simulink model "ProdSys_MakeToStockPULL_CONWIP"  (R2015a)
settings: Solver=ode45  SolverMode=SingleTasking  StartTime=0.0  StopTime=10.0  RelTol=1e-3
undefined symbols (not defined in the file or in its folder): se_randomizeseeds
libraries: simeventslib x10, simulink x1
(part 1 of 2)
settings Model: CovSFcnEnable=off  Creator=AnotherUser  LastModifiedBy=gthiers3
settings OptimizationCC: BlockReduction=off  BooleanDataType=off
settings DebuggingCC: SaveWithParameterizedLinksMsg=none  UnderspecifiedInitializationDetection=Classic  MergeDetectMultiDrivingBlocksExec=none  SignalResolutionControl=TryResolveAllWithWarning  StrictBusMsg=Warning
settings HardwareCC: TargetUnknown=on

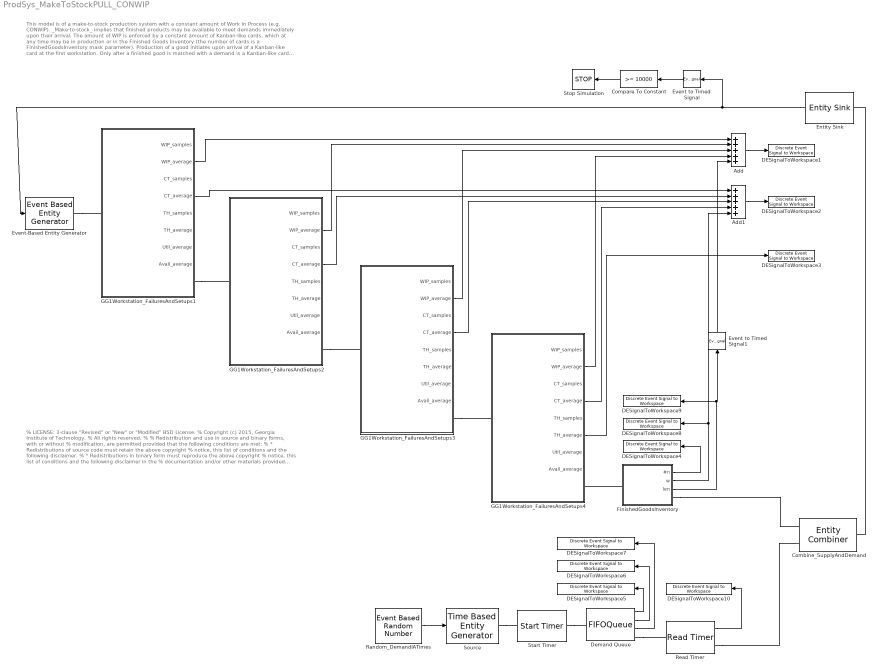
== system ProdSys_MakeToStockPULL_CONWIP ==
  note: This model is of a make-to-stock production system with a constant amount of Work In Process (e.g. CONWIP).
      | _Make-to-stock_ implies that finished products may be available to meet demands immediately upon their arrival.
      | The amount of WIP is enforced by a constant amount of Kanban-like cards, which at any time may be in production
      | or in the Finished Goods Inventory (the number of cards is a FinishedGoodsInventory mask parameter). Production
      | of a good initiates upon arrival of a Kanban-like card at the first workstation.  Only after a finished good is matched
      | with a demand is a Kanban-like card freed and recycled through a feedback loop.
      |
      | NOTE that each GG1Workstation_FailuresAndSetups# is a usage of a block in the SingleWorkstationModelLibrary,
      | and that library may need to be accessible on MATLAB's path.
  note: % LICENSE: 3-clause "Revised" or "New" or "Modified" BSD License.
      | % Copyright (c) 2015, Georgia Institute of Technology.
      | % All rights reserved.
      | %
      | % Redistribution and use in source and binary forms, with or without
      | % modification, are permitted provided that the following conditions are met:
      | % * Redistributions of source code must retain the above copyright
      | % notice, this list of conditions and the following disclaimer.
      | % * Redistributions in binary form must reproduce the above copyright
      | % notice, this list of conditions and the following disclaimer in the
      | % documentation and/or other materials provided with the distribution.
      | % * Neither the name of the Georgia Institute of Technology nor the
      | % names of its contributors may be used to endorse or promote products
      | % derived from this software without specific prior written permission.
      | %
      | % THIS SOFTWARE IS PROVIDED BY THE COPYRIGHT HOLDERS AND CONTRIBUTORS "AS IS" AND
      | % ANY EXPRESS OR IMPLIED WARRANTIES, INCLUDING, BUT NOT LIMITED TO, THE IMPLIED
      | % WARRANTIES OF MERCHANTABILITY AND FITNESS FOR A PARTICULAR PURPOSE ARE
      | % DISCLAIMED. IN NO EVENT SHALL THE GEORGIA INSTITUTE OF TECHNOLOGY BE LIABLE FOR
      | % ANY DIRECT, INDIRECT, INCIDENTAL, SPECIAL, EXEMPLARY, OR CONSEQUENTIAL DAMAGES
      | % (INCLUDING, BUT NOT LIMITED TO, PROCUREMENT OF SUBSTITUTE GOODS OR SERVICES;
      | % LOSS OF USE, DATA, OR PROFITS; OR BUSINESS INTERRUPTION) HOWEVER CAUSED AND
      | % ON ANY THEORY OF LIABILITY, WHETHER IN CONTRACT, STRICT LIABILITY, OR TORT
      | % (INCLUDING NEGLIGENCE OR OTHERWISE) ARISING IN ANY WAY OUT OF THE USE OF THIS
      | % SOFTWARE, EVEN IF ADVISED OF THE POSSIBILITY OF SUCH DAMAGE.
  Add : Sum  Inputs=+++++
  Add1 : Sum  Inputs=+++++
  Combine_SupplyAndDemand : EntityCombiner  NumberInputPorts=2  RetainComponentEntities=off
  Compare To Constant : simulink/Logic and Bit Operations/Compare To Constant  relop=>=  const=10000  OutDataTypeStr=boolean
  DESignalToWorkspace1 : simeventslib/SimEvents Sinks/Discrete Event Signal to Workspace  VariableName=WIP_average  SaveFormat=Structure With Time  isMonitorOnly=off  isRecordIC=off
  DESignalToWorkspace10 : simeventslib/SimEvents Sinks/Discrete Event Signal to Workspace  VariableName=DemandWaitTimes  SaveFormat=Structure With Time  isMonitorOnly=off  isRecordIC=off
  DESignalToWorkspace2 : simeventslib/SimEvents Sinks/Discrete Event Signal to Workspace  VariableName=CT_average  SaveFormat=Structure With Time  isMonitorOnly=off  isRecordIC=off
  DESignalToWorkspace3 : simeventslib/SimEvents Sinks/Discrete Event Signal to Workspace  VariableName=TH_average  SaveFormat=Structure With Time  isMonitorOnly=off  isRecordIC=off
  DESignalToWorkspace4 : simeventslib/SimEvents Sinks/Discrete Event Signal to Workspace  VariableName=FGI_samples  SaveFormat=Structure With Time  isMonitorOnly=off  isRecordIC=off
  DESignalToWorkspace5 : simeventslib/SimEvents Sinks/Discrete Event Signal to Workspace  VariableName=Backorders_samples  SaveFormat=Structure With Time  isMonitorOnly=off  isRecordIC=off
  DESignalToWorkspace6 : simeventslib/SimEvents Sinks/Discrete Event Signal to Workspace  VariableName=Backorders_avgWait  SaveFormat=Structure With Time  isMonitorOnly=off  isRecordIC=off
  DESignalToWorkspace7 : simeventslib/SimEvents Sinks/Discrete Event Signal to Workspace  VariableName=Backorders_avgLen  SaveFormat=Structure With Time  isMonitorOnly=off  isRecordIC=off
  DESignalToWorkspace8 : simeventslib/SimEvents Sinks/Discrete Event Signal to Workspace  VariableName=FGI_avgWait  SaveFormat=Structure With Time  isMonitorOnly=off  isRecordIC=off
  DESignalToWorkspace9 : simeventslib/SimEvents Sinks/Discrete Event Signal to Workspace  VariableName=FGI_avgLen  SaveFormat=Structure With Time  isMonitorOnly=off  isRecordIC=off
  Demand Queue : FIFOQueue  Capacity=inf  StatNumberInBlock=on  StatAverageWait=on  StatAverageQueueLength=on
      settings: OutputPortMap=o1,o2,o3
  Entity Sink : EntitySink  StatNumberArrived=on
  Event to Timed Signal : EventToTimedSignal
  Event to Timed Signal1 : EventToTimedSignal
  Event-Based Entity Generator : EventBasedEntityGenerator  ResponseDuringBlockage=Delay first pending entity
  FinishedGoodsInventory : Subsystem  mask{NumberOfEventsPerPeriod=10}
      mask prompts: NumberOfEventsPerPeriod "Number of Kanban-like cards in the system:"
      mask TypeOptions NumberOfEventsPerPeriod: T0_FcnCallGen/NumberOfEventsPerPeriod
      mask DialogControl DescTextVar Prompt: Finished Goods Inventory:  Make-to-stock implies that finished goods may be produced in advance of demand arrivals.  This subsystem is effectively a queue, storing finished goods which have not yet been matched with demand.
  GG1Workstation_FailuresAndSetups1 : Subsystem  InitFcn=se_randomizeseeds(gcs, 'Mode', 'All')
      settings: CopyFcn=set_param(gcb, 'LinkStatus', 'none');
  GG1Workstation_FailuresAndSetups2 : Subsystem  InitFcn=se_randomizeseeds(gcs, 'Mode', 'All')
      settings: CopyFcn=set_param(gcb, 'LinkStatus', 'none');
  GG1Workstation_FailuresAndSetups3 : Subsystem  InitFcn=se_randomizeseeds(gcs, 'Mode', 'All')
      settings: CopyFcn=set_param(gcb, 'LinkStatus', 'none');
  GG1Workstation_FailuresAndSetups4 : Subsystem  InitFcn=se_randomizeseeds(gcs, 'Mode', 'All')
      settings: CopyFcn=set_param(gcb, 'LinkStatus', 'none');
  Random_DemandIATimes : EventBasedRandomNumber  Distribution=Gamma  scaleGam=2  shapeGam=10  meanNorm=100  stdNorm=eps  Seed=10339
  Read Timer : ReadTimer  StatTimeElapsed=on
      settings: OutputPortMap=o2
  Source : TimeBasedEntityGenerator  GenerateEntitiesUpon=Intergeneration time from port t
  Start Timer : StartTimer
  Stop Simulation : Stop
  wires:
  Random_DemandIATimes/1 -> Source/1
  Entity Sink/1 -> Event to Timed Signal/1, Event-Based Entity Generator/1
  Compare To Constant/1 -> Stop Simulation/1
  Event to Timed Signal/1 -> Compare To Constant/1
  GG1Workstation_FailuresAndSetups1/2(WIP_average) -> Add/1
  GG1Workstation_FailuresAndSetups4/6(TH_average) -> DESignalToWorkspace3/1
  GG1Workstation_FailuresAndSetups1/4(CT_average) -> Add1/1
  GG1Workstation_FailuresAndSetups2/4(CT_average) -> Add1/2
  GG1Workstation_FailuresAndSetups3/4(CT_average) -> Add1/3
  GG1Workstation_FailuresAndSetups4/4(CT_average) -> Add1/4
  GG1Workstation_FailuresAndSetups2/2(WIP_average) -> Add/2
  GG1Workstation_FailuresAndSetups3/2(WIP_average) -> Add/3
  GG1Workstation_FailuresAndSetups4/2(WIP_average) -> Add/4
  Add/1 -> DESignalToWorkspace1/1
  Add1/1 -> DESignalToWorkspace2/1
  FinishedGoodsInventory/1(#n) -> DESignalToWorkspace4/1
  Demand Queue/1 -> DESignalToWorkspace5/1
  Demand Queue/2 -> DESignalToWorkspace6/1
  Demand Queue/3 -> DESignalToWorkspace7/1
  FinishedGoodsInventory/3(len) -> DESignalToWorkspace9/1, Event to Timed Signal1/1
  Read Timer/1 -> DESignalToWorkspace10/1
  FinishedGoodsInventory/2(w) -> Add1/5, DESignalToWorkspace8/1
  Event to Timed Signal1/1 -> Add/5
  connections:
  Source/RConn1 -- Start Timer/LConn1
  FinishedGoodsInventory/LConn1 -- GG1Workstation_FailuresAndSetups4/RConn1
  GG1Workstation_FailuresAndSetups3/RConn1 -- GG1Workstation_FailuresAndSetups4/LConn1
  GG1Workstation_FailuresAndSetups2/RConn1 -- GG1Workstation_FailuresAndSetups3/LConn1
  GG1Workstation_FailuresAndSetups1/RConn1 -- GG1Workstation_FailuresAndSetups2/LConn1
  Event-Based Entity Generator/RConn1 -- GG1Workstation_FailuresAndSetups1/LConn1
  FinishedGoodsInventory/RConn1 -- Combine_SupplyAndDemand/LConn1
  Combine_SupplyAndDemand/RConn1 -- Entity Sink/LConn1
  Start Timer/RConn1 -- Demand Queue/LConn1
  Demand Queue/RConn1 -- Read Timer/LConn1
  Read Timer/RConn1 -- Combine_SupplyAndDemand/LConn2

== system ProdSys_MakeToStockPULL_CONWIP/FinishedGoodsInventory ==
  FIFO Queue : FIFOQueue  Capacity=inf  StatNumberInBlock=on  StatAverageWait=on  StatAverageQueueLength=on
      settings: OutputPortMap=o1,o2,o3
  Path Combiner : PathCombiner  NumberInputPorts=2
  T0_EntityGen : EventBasedEntityGenerator  GenerateEntitiesUpon=Function call from port fcn
  T0_FcnCallGen : TimeBasedFunctionCallGenerator  EventGenerationMode=Only at simulation start  NumberOfEventsPerPeriod=NumberOfEventsPerPeriod
  IN : PMIOPort  Port=1  Side=Left
  OUT : PMIOPort  Port=2  Side=Right
  #n : Outport
  w : Outport  Port=2
  len : Outport  Port=3
  wires:
  T0_FcnCallGen/1 -> T0_EntityGen/1
  FIFO Queue/1 -> #n/1
  FIFO Queue/2 -> w/1
  FIFO Queue/3 -> len/1
  connections:
  T0_EntityGen/RConn1 -- Path Combiner/LConn1
  Path Combiner/RConn1 -- FIFO Queue/LConn1
  IN/RConn1 -- Path Combiner/LConn2
  OUT/RConn1 -- FIFO Queue/RConn1

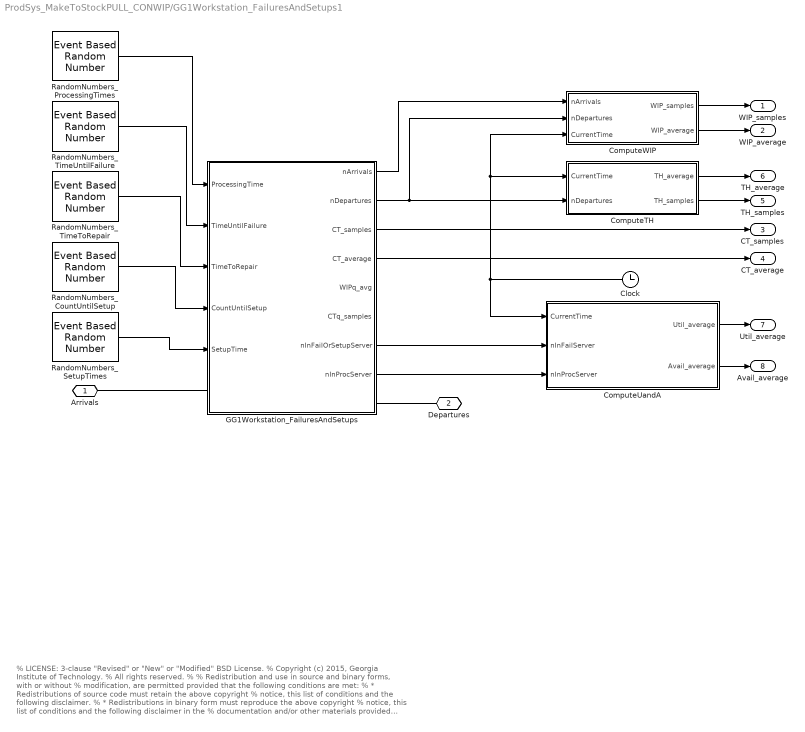
== system ProdSys_MakeToStockPULL_CONWIP/GG1Workstation_FailuresAndSetups1 ==
  note: % LICENSE: 3-clause "Revised" or "New" or "Modified" BSD License.
      | % Copyright (c) 2015, Georgia Institute of Technology.
      | % All rights reserved.
      | %
      | % Redistribution and use in source and binary forms, with or without
      | % modification, are permitted provided that the following conditions are met:
      | % * Redistributions of source code must retain the above copyright
      | % notice, this list of conditions and the following disclaimer.
      | % * Redistributions in binary form must reproduce the above copyright
      | % notice, this list of conditions and the following disclaimer in the
      | % documentation and/or other materials provided with the distribution.
      | % * Neither the name of the Georgia Institute of Technology nor the
      | % names of its contributors may be used to endorse or promote products
      | % derived from this software without specific prior written permission.
      | %
      | % THIS SOFTWARE IS PROVIDED BY THE COPYRIGHT HOLDERS AND CONTRIBUTORS "AS IS" AND
      | % ANY EXPRESS OR IMPLIED WARRANTIES, INCLUDING, BUT NOT LIMITED TO, THE IMPLIED
      | % WARRANTIES OF MERCHANTABILITY AND FITNESS FOR A PARTICULAR PURPOSE ARE
      | % DISCLAIMED. IN NO EVENT SHALL THE GEORGIA INSTITUTE OF TECHNOLOGY BE LIABLE FOR
      | % ANY DIRECT, INDIRECT, INCIDENTAL, SPECIAL, EXEMPLARY, OR CONSEQUENTIAL DAMAGES
      | % (INCLUDING, BUT NOT LIMITED TO, PROCUREMENT OF SUBSTITUTE GOODS OR SERVICES;
      | % LOSS OF USE, DATA, OR PROFITS; OR BUSINESS INTERRUPTION) HOWEVER CAUSED AND
      | % ON ANY THEORY OF LIABILITY, WHETHER IN CONTRACT, STRICT LIABILITY, OR TORT
      | % (INCLUDING NEGLIGENCE OR OTHERWISE) ARISING IN ANY WAY OUT OF THE USE OF THIS
      | % SOFTWARE, EVEN IF ADVISED OF THE POSSIBILITY OF SUCH DAMAGE.
  Clock : Clock
  ComputeTH : Subsystem
  ComputeUandA : Subsystem
  ComputeWIP : Subsystem
  GG1Workstation_FailuresAndSetups : Subsystem  mask{Capacity=Inf}
      mask prompts: Capacity "Queue Capacity"
      mask TypeOptions Capacity: FIFOQueue/Capacity
      mask DialogControl DescTextVar Prompt: GG1 Workstation, with a random count of entities serviced until a setup, and random setup times.  Setups are functionally equivalent to any non-preemptive (e.g. non-interrupting) downtime, for example preventative maintenance.
  RandomNumbers_CountUntilSetup : EventBasedRandomNumber  Distribution=Gaussian (normal)  meanExp=100  minUnif=40  maxUnif=40  pOneBern=40  pSuccessBino=40  numTrialBino=40  minTri=10  maxTri=10  modeTri=10  scaleGam=166.6667  shapeGam=0.72  meanNorm=2147483647  stdNorm=32  pSuccessGeo=40  meanPoiss=40  thresholdLogn=40  scaleLogn=40  shapeLogn=40  thresholdLogl=40  scaleLogl=40  minBeta=40  maxBeta=40  shape1Beta=40  shape2Beta=40  minUnid=40  maxUnid=40  numValueUnid=40  thresholdWbl=40  scaleWbl=40  shapeWbl=40  valueVecCont=40  cdfVecCont=40  valueVecDisc=40  probVecDisc=40  Seed=9514
  RandomNumbers_ProcessingTimes : EventBasedRandomNumber  Distribution=Gamma  meanExp=75  minUnif=40  maxUnif=40  pOneBern=40  pSuccessBino=40  numTrialBino=40  minTri=40  maxTri=40  modeTri=40  scaleGam=4.2188e-15  shapeGam=4503599627370496  meanNorm=50  stdNorm=eps  pSuccessGeo=40  meanPoiss=40  thresholdLogn=40  scaleLogn=40  shapeLogn=40  thresholdLogl=40  scaleLogl=40  minBeta=40  maxBeta=40  shape1Beta=40  shape2Beta=40  minUnid=40  maxUnid=40  numValueUnid=40  thresholdWbl=40  scaleWbl=40  shapeWbl=40  valueVecCont=40  cdfVecCont=40  valueVecDisc=40  probVecDisc=40  Seed=12731
  RandomNumbers_SetupTimes : EventBasedRandomNumber  Distribution=Gaussian (normal)  meanExp=400  minUnif=40  maxUnif=40  pOneBern=40  pSuccessBino=40  numTrialBino=40  minTri=38  maxTri=38  modeTri=38  scaleGam=20  meanNorm=2.2204e-16  stdNorm=3.3087e-24  pSuccessGeo=40  meanPoiss=40  thresholdLogn=40  scaleLogn=40  shapeLogn=40  thresholdLogl=40  scaleLogl=40  minBeta=40  maxBeta=40  shape1Beta=40  shape2Beta=40  minUnid=40  maxUnid=40  numValueUnid=40  thresholdWbl=40  scaleWbl=40  shapeWbl=40  valueVecCont=40  cdfVecCont=40  probVecDisc=[0 1]  Seed=15948
  RandomNumbers_TimeToRepair : EventBasedRandomNumber  Distribution=Gaussian (normal)  meanExp=400  minUnif=40  maxUnif=40  pOneBern=40  pSuccessBino=40  numTrialBino=40  minTri=38  maxTri=38  modeTri=38  scaleGam=20  meanNorm=2.2204e-16  stdNorm=3.3087e-24  pSuccessGeo=40  meanPoiss=40  thresholdLogn=40  scaleLogn=40  shapeLogn=40  thresholdLogl=40  scaleLogl=40  minBeta=40  maxBeta=40  shape1Beta=40  shape2Beta=40  minUnid=40  maxUnid=40  numValueUnid=40  thresholdWbl=40  scaleWbl=40  shapeWbl=40  valueVecCont=40  cdfVecCont=40  probVecDisc=[0 1]  Seed=19165
  RandomNumbers_TimeUntilFailure : EventBasedRandomNumber  Distribution=Gaussian (normal)  meanExp=2500  minUnif=40  maxUnif=40  pOneBern=40  pSuccessBino=40  numTrialBino=40  minTri=114  maxTri=114  modeTri=114  scaleGam=166.6667  shapeGam=0.72  meanNorm=2147483647  stdNorm=32  pSuccessGeo=40  meanPoiss=40  thresholdLogn=40  scaleLogn=40  shapeLogn=40  thresholdLogl=40  scaleLogl=40  minBeta=40  maxBeta=40  shape1Beta=40  shape2Beta=40  minUnid=40  maxUnid=40  numValueUnid=40  thresholdWbl=40  scaleWbl=40  shapeWbl=40  valueVecCont=40  cdfVecCont=40  valueVecDisc=40  probVecDisc=40  Seed=22382
  Arrivals : PMIOPort  Port=1  Side=Left
  Departures : PMIOPort  Port=2  Side=Right
  WIP_samples : Outport
  WIP_average : Outport  Port=2
  CT_samples : Outport  Port=3
  CT_average : Outport  Port=4
  TH_samples : Outport  Port=5
  TH_average : Outport  Port=6
  Util_average : Outport  Port=7
  Avail_average : Outport  Port=8
  wires:
  ComputeUandA/2(Avail_average) -> Avail_average/1
  ComputeUandA/1(Util_average) -> Util_average/1
  GG1Workstation_FailuresAndSetups/8(nInProcServer) -> ComputeUandA/3(nInProcServer)
  GG1Workstation_FailuresAndSetups/7(nInFailOrSetupServer) -> ComputeUandA/2(nInFailServer)
  RandomNumbers_SetupTimes/1 -> GG1Workstation_FailuresAndSetups/5(SetupTime)
  RandomNumbers_CountUntilSetup/1 -> GG1Workstation_FailuresAndSetups/4(CountUntilSetup)
  RandomNumbers_TimeToRepair/1 -> GG1Workstation_FailuresAndSetups/3(TimeToRepair)
  RandomNumbers_TimeUntilFailure/1 -> GG1Workstation_FailuresAndSetups/2(TimeUntilFailure)
  ComputeTH/2(TH_samples) -> TH_samples/1
  ComputeTH/1(TH_average) -> TH_average/1
  Clock/1 -> ComputeUandA/1(CurrentTime), ComputeTH/1(CurrentTime), ComputeWIP/3(CurrentTime)
  GG1Workstation_FailuresAndSetups/1(nArrivals) -> ComputeWIP/1(nArrivals)
  ComputeWIP/2(WIP_average) -> WIP_average/1
  ComputeWIP/1(WIP_samples) -> WIP_samples/1
  GG1Workstation_FailuresAndSetups/4(CT_average) -> CT_average/1
  GG1Workstation_FailuresAndSetups/3(CT_samples) -> CT_samples/1
  GG1Workstation_FailuresAndSetups/2(nDepartures) -> ComputeTH/2(nDepartures), ComputeWIP/2(nDepartures)
  RandomNumbers_ProcessingTimes/1 -> GG1Workstation_FailuresAndSetups/1(ProcessingTime)
  connections:
  Arrivals/RConn1 -- GG1Workstation_FailuresAndSetups/LConn1
  GG1Workstation_FailuresAndSetups/RConn1 -- Departures/RConn1

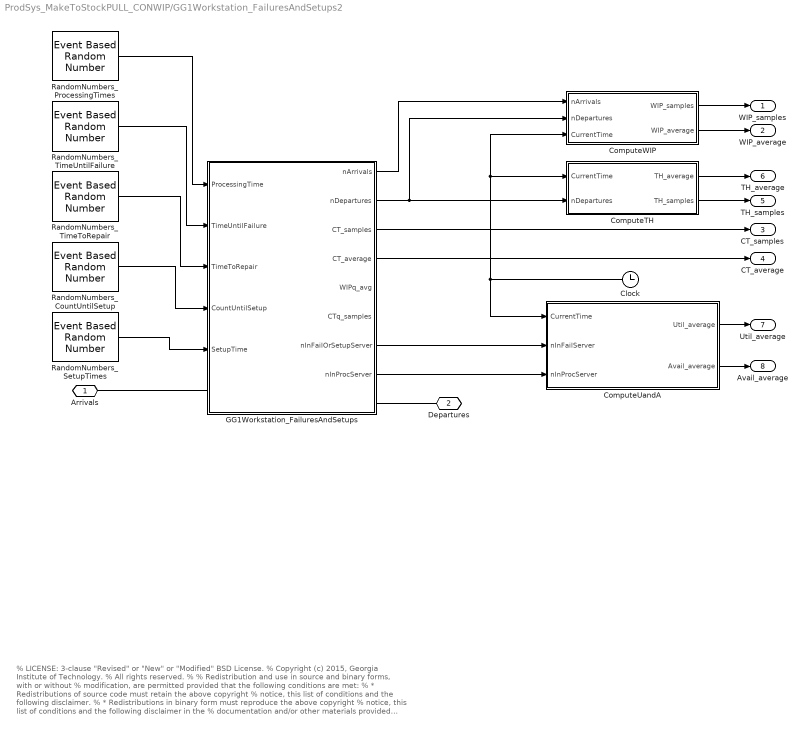
== system ProdSys_MakeToStockPULL_CONWIP/GG1Workstation_FailuresAndSetups2 ==
  note: % LICENSE: 3-clause "Revised" or "New" or "Modified" BSD License.
      | % Copyright (c) 2015, Georgia Institute of Technology.
      | % All rights reserved.
      | %
      | % Redistribution and use in source and binary forms, with or without
      | % modification, are permitted provided that the following conditions are met:
      | % * Redistributions of source code must retain the above copyright
      | % notice, this list of conditions and the following disclaimer.
      | % * Redistributions in binary form must reproduce the above copyright
      | % notice, this list of conditions and the following disclaimer in the
      | % documentation and/or other materials provided with the distribution.
      | % * Neither the name of the Georgia Institute of Technology nor the
      | % names of its contributors may be used to endorse or promote products
      | % derived from this software without specific prior written permission.
      | %
      | % THIS SOFTWARE IS PROVIDED BY THE COPYRIGHT HOLDERS AND CONTRIBUTORS "AS IS" AND
      | % ANY EXPRESS OR IMPLIED WARRANTIES, INCLUDING, BUT NOT LIMITED TO, THE IMPLIED
      | % WARRANTIES OF MERCHANTABILITY AND FITNESS FOR A PARTICULAR PURPOSE ARE
      | % DISCLAIMED. IN NO EVENT SHALL THE GEORGIA INSTITUTE OF TECHNOLOGY BE LIABLE FOR
      | % ANY DIRECT, INDIRECT, INCIDENTAL, SPECIAL, EXEMPLARY, OR CONSEQUENTIAL DAMAGES
      | % (INCLUDING, BUT NOT LIMITED TO, PROCUREMENT OF SUBSTITUTE GOODS OR SERVICES;
      | % LOSS OF USE, DATA, OR PROFITS; OR BUSINESS INTERRUPTION) HOWEVER CAUSED AND
      | % ON ANY THEORY OF LIABILITY, WHETHER IN CONTRACT, STRICT LIABILITY, OR TORT
      | % (INCLUDING NEGLIGENCE OR OTHERWISE) ARISING IN ANY WAY OUT OF THE USE OF THIS
      | % SOFTWARE, EVEN IF ADVISED OF THE POSSIBILITY OF SUCH DAMAGE.
  Clock : Clock
  ComputeTH : Subsystem
  ComputeUandA : Subsystem
  ComputeWIP : Subsystem
  GG1Workstation_FailuresAndSetups : Subsystem  mask{Capacity=Inf}
      mask prompts: Capacity "Queue Capacity"
      mask TypeOptions Capacity: FIFOQueue/Capacity
      mask DialogControl DescTextVar Prompt: GG1 Workstation, with a random count of entities serviced until a setup, and random setup times.  Setups are functionally equivalent to any non-preemptive (e.g. non-interrupting) downtime, for example preventative maintenance.
  RandomNumbers_CountUntilSetup : EventBasedRandomNumber  Distribution=Gaussian (normal)  meanExp=100  minUnif=40  maxUnif=40  pOneBern=40  pSuccessBino=40  numTrialBino=40  minTri=10  maxTri=10  modeTri=10  scaleGam=166.6667  shapeGam=0.72  meanNorm=2147483647  stdNorm=32  pSuccessGeo=40  meanPoiss=40  thresholdLogn=40  scaleLogn=40  shapeLogn=40  thresholdLogl=40  scaleLogl=40  minBeta=40  maxBeta=40  shape1Beta=40  shape2Beta=40  minUnid=40  maxUnid=40  numValueUnid=40  thresholdWbl=40  scaleWbl=40  shapeWbl=40  valueVecCont=40  cdfVecCont=40  valueVecDisc=40  probVecDisc=40  Seed=25599
  RandomNumbers_ProcessingTimes : EventBasedRandomNumber  Distribution=Gamma  meanExp=75  minUnif=40  maxUnif=40  pOneBern=40  pSuccessBino=40  numTrialBino=40  minTri=40  maxTri=40  modeTri=40  scaleGam=4.2188e-15  shapeGam=4503599627370496  meanNorm=50  stdNorm=eps  pSuccessGeo=40  meanPoiss=40  thresholdLogn=40  scaleLogn=40  shapeLogn=40  thresholdLogl=40  scaleLogl=40  minBeta=40  maxBeta=40  shape1Beta=40  shape2Beta=40  minUnid=40  maxUnid=40  numValueUnid=40  thresholdWbl=40  scaleWbl=40  shapeWbl=40  valueVecCont=40  cdfVecCont=40  valueVecDisc=40  probVecDisc=40  Seed=28816
  RandomNumbers_SetupTimes : EventBasedRandomNumber  Distribution=Gaussian (normal)  meanExp=400  minUnif=40  maxUnif=40  pOneBern=40  pSuccessBino=40  numTrialBino=40  minTri=38  maxTri=38  modeTri=38  scaleGam=20  meanNorm=2.2204e-16  stdNorm=3.3087e-24  pSuccessGeo=40  meanPoiss=40  thresholdLogn=40  scaleLogn=40  shapeLogn=40  thresholdLogl=40  scaleLogl=40  minBeta=40  maxBeta=40  shape1Beta=40  shape2Beta=40  minUnid=40  maxUnid=40  numValueUnid=40  thresholdWbl=40  scaleWbl=40  shapeWbl=40  valueVecCont=40  cdfVecCont=40  probVecDisc=[0 1]  Seed=32033
  RandomNumbers_TimeToRepair : EventBasedRandomNumber  Distribution=Gaussian (normal)  meanExp=400  minUnif=40  maxUnif=40  pOneBern=40  pSuccessBino=40  numTrialBino=40  minTri=38  maxTri=38  modeTri=38  scaleGam=20  meanNorm=2.2204e-16  stdNorm=3.3087e-24  pSuccessGeo=40  meanPoiss=40  thresholdLogn=40  scaleLogn=40  shapeLogn=40  thresholdLogl=40  scaleLogl=40  minBeta=40  maxBeta=40  shape1Beta=40  shape2Beta=40  minUnid=40  maxUnid=40  numValueUnid=40  thresholdWbl=40  scaleWbl=40  shapeWbl=40  valueVecCont=40  cdfVecCont=40  probVecDisc=[0 1]  Seed=35250
  RandomNumbers_TimeUntilFailure : EventBasedRandomNumber  Distribution=Gaussian (normal)  meanExp=2500  minUnif=40  maxUnif=40  pOneBern=40  pSuccessBino=40  numTrialBino=40  minTri=114  maxTri=114  modeTri=114  scaleGam=166.6667  shapeGam=0.72  meanNorm=2147483647  stdNorm=32  pSuccessGeo=40  meanPoiss=40  thresholdLogn=40  scaleLogn=40  shapeLogn=40  thresholdLogl=40  scaleLogl=40  minBeta=40  maxBeta=40  shape1Beta=40  shape2Beta=40  minUnid=40  maxUnid=40  numValueUnid=40  thresholdWbl=40  scaleWbl=40  shapeWbl=40  valueVecCont=40  cdfVecCont=40  valueVecDisc=40  probVecDisc=40  Seed=38467
  Arrivals : PMIOPort  Port=1  Side=Left
  Departures : PMIOPort  Port=2  Side=Right
  WIP_samples : Outport
  WIP_average : Outport  Port=2
  CT_samples : Outport  Port=3
  CT_average : Outport  Port=4
  TH_samples : Outport  Port=5
  TH_average : Outport  Port=6
  Util_average : Outport  Port=7
  Avail_average : Outport  Port=8
  wires:
  ComputeUandA/2(Avail_average) -> Avail_average/1
  ComputeUandA/1(Util_average) -> Util_average/1
  GG1Workstation_FailuresAndSetups/8(nInProcServer) -> ComputeUandA/3(nInProcServer)
  GG1Workstation_FailuresAndSetups/7(nInFailOrSetupServer) -> ComputeUandA/2(nInFailServer)
  RandomNumbers_SetupTimes/1 -> GG1Workstation_FailuresAndSetups/5(SetupTime)
  RandomNumbers_CountUntilSetup/1 -> GG1Workstation_FailuresAndSetups/4(CountUntilSetup)
  RandomNumbers_TimeToRepair/1 -> GG1Workstation_FailuresAndSetups/3(TimeToRepair)
  RandomNumbers_TimeUntilFailure/1 -> GG1Workstation_FailuresAndSetups/2(TimeUntilFailure)
  ComputeTH/2(TH_samples) -> TH_samples/1
  ComputeTH/1(TH_average) -> TH_average/1
  Clock/1 -> ComputeUandA/1(CurrentTime), ComputeTH/1(CurrentTime), ComputeWIP/3(CurrentTime)
  GG1Workstation_FailuresAndSetups/1(nArrivals) -> ComputeWIP/1(nArrivals)
  ComputeWIP/2(WIP_average) -> WIP_average/1
  ComputeWIP/1(WIP_samples) -> WIP_samples/1
  GG1Workstation_FailuresAndSetups/4(CT_average) -> CT_average/1
  GG1Workstation_FailuresAndSetups/3(CT_samples) -> CT_samples/1
  GG1Workstation_FailuresAndSetups/2(nDepartures) -> ComputeTH/2(nDepartures), ComputeWIP/2(nDepartures)
  RandomNumbers_ProcessingTimes/1 -> GG1Workstation_FailuresAndSetups/1(ProcessingTime)
  connections:
  Arrivals/RConn1 -- GG1Workstation_FailuresAndSetups/LConn1
  GG1Workstation_FailuresAndSetups/RConn1 -- Departures/RConn1

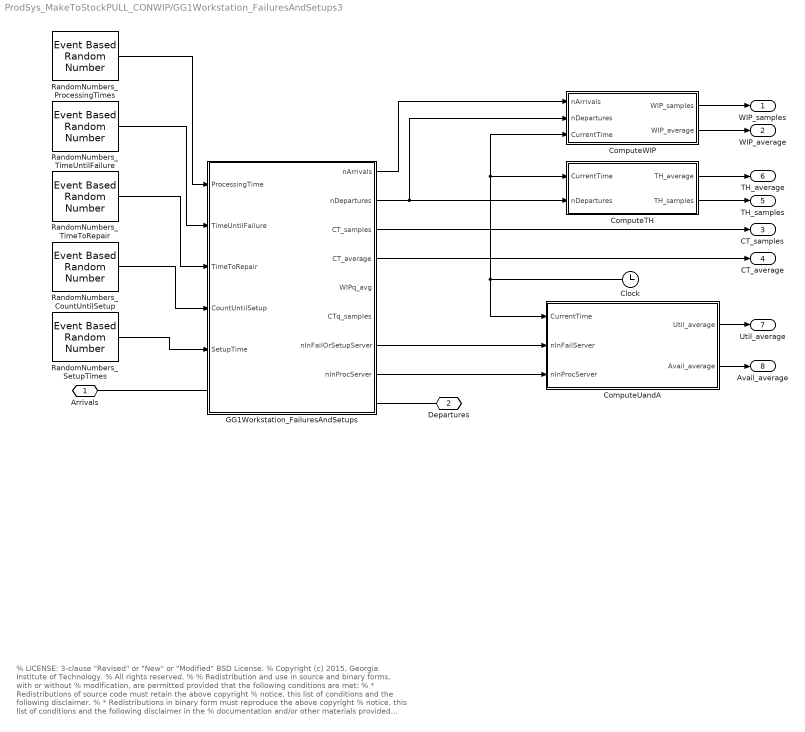
== system ProdSys_MakeToStockPULL_CONWIP/GG1Workstation_FailuresAndSetups3 ==
  note: % LICENSE: 3-clause "Revised" or "New" or "Modified" BSD License.
      | % Copyright (c) 2015, Georgia Institute of Technology.
      | % All rights reserved.
      | %
      | % Redistribution and use in source and binary forms, with or without
      | % modification, are permitted provided that the following conditions are met:
      | % * Redistributions of source code must retain the above copyright
      | % notice, this list of conditions and the following disclaimer.
      | % * Redistributions in binary form must reproduce the above copyright
      | % notice, this list of conditions and the following disclaimer in the
      | % documentation and/or other materials provided with the distribution.
      | % * Neither the name of the Georgia Institute of Technology nor the
      | % names of its contributors may be used to endorse or promote products
      | % derived from this software without specific prior written permission.
      | %
      | % THIS SOFTWARE IS PROVIDED BY THE COPYRIGHT HOLDERS AND CONTRIBUTORS "AS IS" AND
      | % ANY EXPRESS OR IMPLIED WARRANTIES, INCLUDING, BUT NOT LIMITED TO, THE IMPLIED
      | % WARRANTIES OF MERCHANTABILITY AND FITNESS FOR A PARTICULAR PURPOSE ARE
      | % DISCLAIMED. IN NO EVENT SHALL THE GEORGIA INSTITUTE OF TECHNOLOGY BE LIABLE FOR
      | % ANY DIRECT, INDIRECT, INCIDENTAL, SPECIAL, EXEMPLARY, OR CONSEQUENTIAL DAMAGES
      | % (INCLUDING, BUT NOT LIMITED TO, PROCUREMENT OF SUBSTITUTE GOODS OR SERVICES;
      | % LOSS OF USE, DATA, OR PROFITS; OR BUSINESS INTERRUPTION) HOWEVER CAUSED AND
      | % ON ANY THEORY OF LIABILITY, WHETHER IN CONTRACT, STRICT LIABILITY, OR TORT
      | % (INCLUDING NEGLIGENCE OR OTHERWISE) ARISING IN ANY WAY OUT OF THE USE OF THIS
      | % SOFTWARE, EVEN IF ADVISED OF THE POSSIBILITY OF SUCH DAMAGE.
  Clock : Clock
  ComputeTH : Subsystem
  ComputeUandA : Subsystem
  ComputeWIP : Subsystem
  GG1Workstation_FailuresAndSetups : Subsystem  mask{Capacity=Inf}
      mask prompts: Capacity "Queue Capacity"
      mask TypeOptions Capacity: FIFOQueue/Capacity
      mask DialogControl DescTextVar Prompt: GG1 Workstation, with a random count of entities serviced until a setup, and random setup times.  Setups are functionally equivalent to any non-preemptive (e.g. non-interrupting) downtime, for example preventative maintenance.
  RandomNumbers_CountUntilSetup : EventBasedRandomNumber  Distribution=Gaussian (normal)  meanExp=100  minUnif=40  maxUnif=40  pOneBern=40  pSuccessBino=40  numTrialBino=40  minTri=10  maxTri=10  modeTri=10  scaleGam=166.6667  shapeGam=0.72  meanNorm=2147483647  stdNorm=32  pSuccessGeo=40  meanPoiss=40  thresholdLogn=40  scaleLogn=40  shapeLogn=40  thresholdLogl=40  scaleLogl=40  minBeta=40  maxBeta=40  shape1Beta=40  shape2Beta=40  minUnid=40  maxUnid=40  numValueUnid=40  thresholdWbl=40  scaleWbl=40  shapeWbl=40  valueVecCont=40  cdfVecCont=40  valueVecDisc=40  probVecDisc=40  Seed=41684
  RandomNumbers_ProcessingTimes : EventBasedRandomNumber  Distribution=Gamma  meanExp=75  minUnif=40  maxUnif=40  pOneBern=40  pSuccessBino=40  numTrialBino=40  minTri=40  maxTri=40  modeTri=40  scaleGam=4.2188e-15  shapeGam=4503599627370496  meanNorm=50  stdNorm=eps  pSuccessGeo=40  meanPoiss=40  thresholdLogn=40  scaleLogn=40  shapeLogn=40  thresholdLogl=40  scaleLogl=40  minBeta=40  maxBeta=40  shape1Beta=40  shape2Beta=40  minUnid=40  maxUnid=40  numValueUnid=40  thresholdWbl=40  scaleWbl=40  shapeWbl=40  valueVecCont=40  cdfVecCont=40  valueVecDisc=40  probVecDisc=40  Seed=44901
  RandomNumbers_SetupTimes : EventBasedRandomNumber  Distribution=Gaussian (normal)  meanExp=400  minUnif=40  maxUnif=40  pOneBern=40  pSuccessBino=40  numTrialBino=40  minTri=38  maxTri=38  modeTri=38  scaleGam=20  meanNorm=2.2204e-16  stdNorm=3.3087e-24  pSuccessGeo=40  meanPoiss=40  thresholdLogn=40  scaleLogn=40  shapeLogn=40  thresholdLogl=40  scaleLogl=40  minBeta=40  maxBeta=40  shape1Beta=40  shape2Beta=40  minUnid=40  maxUnid=40  numValueUnid=40  thresholdWbl=40  scaleWbl=40  shapeWbl=40  valueVecCont=40  cdfVecCont=40  probVecDisc=[0 1]  Seed=48118
  RandomNumbers_TimeToRepair : EventBasedRandomNumber  Distribution=Gaussian (normal)  meanExp=400  minUnif=40  maxUnif=40  pOneBern=40  pSuccessBino=40  numTrialBino=40  minTri=38  maxTri=38  modeTri=38  scaleGam=20  meanNorm=2.2204e-16  stdNorm=3.3087e-24  pSuccessGeo=40  meanPoiss=40  thresholdLogn=40  scaleLogn=40  shapeLogn=40  thresholdLogl=40  scaleLogl=40  minBeta=40  maxBeta=40  shape1Beta=40  shape2Beta=40  minUnid=40  maxUnid=40  numValueUnid=40  thresholdWbl=40  scaleWbl=40  shapeWbl=40  valueVecCont=40  cdfVecCont=40  probVecDisc=[0 1]  Seed=53356
  RandomNumbers_TimeUntilFailure : EventBasedRandomNumber  Distribution=Gaussian (normal)  meanExp=2500  minUnif=40  maxUnif=40  pOneBern=40  pSuccessBino=40  numTrialBino=40  minTri=114  maxTri=114  modeTri=114  scaleGam=166.6667  shapeGam=0.72  meanNorm=2147483647  stdNorm=32  pSuccessGeo=40  meanPoiss=40  thresholdLogn=40  scaleLogn=40  shapeLogn=40  thresholdLogl=40  scaleLogl=40  minBeta=40  maxBeta=40  shape1Beta=40  shape2Beta=40  minUnid=40  maxUnid=40  numValueUnid=40  thresholdWbl=40  scaleWbl=40  shapeWbl=40  valueVecCont=40  cdfVecCont=40  valueVecDisc=40  probVecDisc=40  Seed=56573
  Arrivals : PMIOPort  Port=1  Side=Left
  Departures : PMIOPort  Port=2  Side=Right
  WIP_samples : Outport
  WIP_average : Outport  Port=2
  CT_samples : Outport  Port=3
  CT_average : Outport  Port=4
  TH_samples : Outport  Port=5
  TH_average : Outport  Port=6
  Util_average : Outport  Port=7
  Avail_average : Outport  Port=8
  wires:
  ComputeUandA/2(Avail_average) -> Avail_average/1
  ComputeUandA/1(Util_average) -> Util_average/1
  GG1Workstation_FailuresAndSetups/8(nInProcServer) -> ComputeUandA/3(nInProcServer)
  GG1Workstation_FailuresAndSetups/7(nInFailOrSetupServer) -> ComputeUandA/2(nInFailServer)
  RandomNumbers_SetupTimes/1 -> GG1Workstation_FailuresAndSetups/5(SetupTime)
  RandomNumbers_CountUntilSetup/1 -> GG1Workstation_FailuresAndSetups/4(CountUntilSetup)
  RandomNumbers_TimeToRepair/1 -> GG1Workstation_FailuresAndSetups/3(TimeToRepair)
  RandomNumbers_TimeUntilFailure/1 -> GG1Workstation_FailuresAndSetups/2(TimeUntilFailure)
  ComputeTH/2(TH_samples) -> TH_samples/1
  ComputeTH/1(TH_average) -> TH_average/1
  Clock/1 -> ComputeUandA/1(CurrentTime), ComputeTH/1(CurrentTime), ComputeWIP/3(CurrentTime)
  GG1Workstation_FailuresAndSetups/1(nArrivals) -> ComputeWIP/1(nArrivals)
  ComputeWIP/2(WIP_average) -> WIP_average/1
  ComputeWIP/1(WIP_samples) -> WIP_samples/1
  GG1Workstation_FailuresAndSetups/4(CT_average) -> CT_average/1
  GG1Workstation_FailuresAndSetups/3(CT_samples) -> CT_samples/1
  GG1Workstation_FailuresAndSetups/2(nDepartures) -> ComputeTH/2(nDepartures), ComputeWIP/2(nDepartures)
  RandomNumbers_ProcessingTimes/1 -> GG1Workstation_FailuresAndSetups/1(ProcessingTime)
  connections:
  Arrivals/RConn1 -- GG1Workstation_FailuresAndSetups/LConn1
  GG1Workstation_FailuresAndSetups/RConn1 -- Departures/RConn1

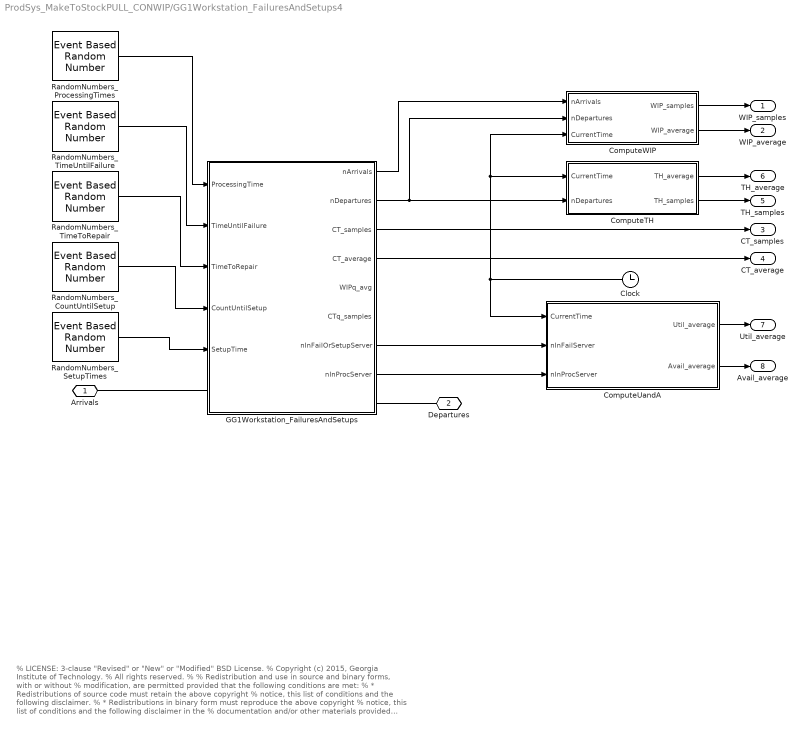
== system ProdSys_MakeToStockPULL_CONWIP/GG1Workstation_FailuresAndSetups4 ==
  note: % LICENSE: 3-clause "Revised" or "New" or "Modified" BSD License.
      | % Copyright (c) 2015, Georgia Institute of Technology.
      | % All rights reserved.
      | %
      | % Redistribution and use in source and binary forms, with or without
      | % modification, are permitted provided that the following conditions are met:
      | % * Redistributions of source code must retain the above copyright
      | % notice, this list of conditions and the following disclaimer.
      | % * Redistributions in binary form must reproduce the above copyright
      | % notice, this list of conditions and the following disclaimer in the
      | % documentation and/or other materials provided with the distribution.
      | % * Neither the name of the Georgia Institute of Technology nor the
      | % names of its contributors may be used to endorse or promote products
      | % derived from this software without specific prior written permission.
      | %
      | % THIS SOFTWARE IS PROVIDED BY THE COPYRIGHT HOLDERS AND CONTRIBUTORS "AS IS" AND
      | % ANY EXPRESS OR IMPLIED WARRANTIES, INCLUDING, BUT NOT LIMITED TO, THE IMPLIED
      | % WARRANTIES OF MERCHANTABILITY AND FITNESS FOR A PARTICULAR PURPOSE ARE
      | % DISCLAIMED. IN NO EVENT SHALL THE GEORGIA INSTITUTE OF TECHNOLOGY BE LIABLE FOR
      | % ANY DIRECT, INDIRECT, INCIDENTAL, SPECIAL, EXEMPLARY, OR CONSEQUENTIAL DAMAGES
      | % (INCLUDING, BUT NOT LIMITED TO, PROCUREMENT OF SUBSTITUTE GOODS OR SERVICES;
      | % LOSS OF USE, DATA, OR PROFITS; OR BUSINESS INTERRUPTION) HOWEVER CAUSED AND
      | % ON ANY THEORY OF LIABILITY, WHETHER IN CONTRACT, STRICT LIABILITY, OR TORT
      | % (INCLUDING NEGLIGENCE OR OTHERWISE) ARISING IN ANY WAY OUT OF THE USE OF THIS
      | % SOFTWARE, EVEN IF ADVISED OF THE POSSIBILITY OF SUCH DAMAGE.
  Clock : Clock
  ComputeTH : Subsystem
  ComputeUandA : Subsystem
  ComputeWIP : Subsystem
  GG1Workstation_FailuresAndSetups : Subsystem  mask{Capacity=Inf}
      mask prompts: Capacity "Queue Capacity"
      mask TypeOptions Capacity: FIFOQueue/Capacity
      mask DialogControl DescTextVar Prompt: GG1 Workstation, with a random count of entities serviced until a setup, and random setup times.  Setups are functionally equivalent to any non-preemptive (e.g. non-interrupting) downtime, for example preventative maintenance.
  RandomNumbers_CountUntilSetup : EventBasedRandomNumber  Distribution=Gaussian (normal)  meanExp=100  minUnif=40  maxUnif=40  pOneBern=40  pSuccessBino=40  numTrialBino=40  minTri=10  maxTri=10  modeTri=10  scaleGam=166.6667  shapeGam=0.72  meanNorm=2147483647  stdNorm=32  pSuccessGeo=40  meanPoiss=40  thresholdLogn=40  scaleLogn=40  shapeLogn=40  thresholdLogl=40  scaleLogl=40  minBeta=40  maxBeta=40  shape1Beta=40  shape2Beta=40  minUnid=40  maxUnid=40  numValueUnid=40  thresholdWbl=40  scaleWbl=40  shapeWbl=40  valueVecCont=40  cdfVecCont=40  valueVecDisc=40  probVecDisc=40  Seed=59790
  RandomNumbers_ProcessingTimes : EventBasedRandomNumber  Distribution=Gamma  meanExp=75  minUnif=40  maxUnif=40  pOneBern=40  pSuccessBino=40  numTrialBino=40  minTri=40  maxTri=40  modeTri=40  scaleGam=4.2188e-15  shapeGam=4503599627370496  meanNorm=50  stdNorm=eps  pSuccessGeo=40  meanPoiss=40  thresholdLogn=40  scaleLogn=40  shapeLogn=40  thresholdLogl=40  scaleLogl=40  minBeta=40  maxBeta=40  shape1Beta=40  shape2Beta=40  minUnid=40  maxUnid=40  numValueUnid=40  thresholdWbl=40  scaleWbl=40  shapeWbl=40  valueVecCont=40  cdfVecCont=40  valueVecDisc=40  probVecDisc=40  Seed=63007
  RandomNumbers_SetupTimes : EventBasedRandomNumber  Distribution=Gaussian (normal)  meanExp=400  minUnif=40  maxUnif=40  pOneBern=40  pSuccessBino=40  numTrialBino=40  minTri=38  maxTri=38  modeTri=38  scaleGam=20  meanNorm=2.2204e-16  stdNorm=3.3087e-24  pSuccessGeo=40  meanPoiss=40  thresholdLogn=40  scaleLogn=40  shapeLogn=40  thresholdLogl=40  scaleLogl=40  minBeta=40  maxBeta=40  shape1Beta=40  shape2Beta=40  minUnid=40  maxUnid=40  numValueUnid=40  thresholdWbl=40  scaleWbl=40  shapeWbl=40  valueVecCont=40  cdfVecCont=40  probVecDisc=[0 1]  Seed=688
  RandomNumbers_TimeToRepair : EventBasedRandomNumber  Distribution=Gaussian (normal)  meanExp=400  minUnif=40  maxUnif=40  pOneBern=40  pSuccessBino=40  numTrialBino=40  minTri=38  maxTri=38  modeTri=38  scaleGam=20  meanNorm=2.2204e-16  stdNorm=3.3087e-24  pSuccessGeo=40  meanPoiss=40  thresholdLogn=40  scaleLogn=40  shapeLogn=40  thresholdLogl=40  scaleLogl=40  minBeta=40  maxBeta=40  shape1Beta=40  shape2Beta=40  minUnid=40  maxUnid=40  numValueUnid=40  thresholdWbl=40  scaleWbl=40  shapeWbl=40  valueVecCont=40  cdfVecCont=40  probVecDisc=[0 1]  Seed=3905
  RandomNumbers_TimeUntilFailure : EventBasedRandomNumber  Distribution=Gaussian (normal)  meanExp=2500  minUnif=40  maxUnif=40  pOneBern=40  pSuccessBino=40  numTrialBino=40  minTri=114  maxTri=114  modeTri=114  scaleGam=166.6667  shapeGam=0.72  meanNorm=2147483647  stdNorm=32  pSuccessGeo=40  meanPoiss=40  thresholdLogn=40  scaleLogn=40  shapeLogn=40  thresholdLogl=40  scaleLogl=40  minBeta=40  maxBeta=40  shape1Beta=40  shape2Beta=40  minUnid=40  maxUnid=40  numValueUnid=40  thresholdWbl=40  scaleWbl=40  shapeWbl=40  valueVecCont=40  cdfVecCont=40  valueVecDisc=40  probVecDisc=40  Seed=7122
  Arrivals : PMIOPort  Port=1  Side=Left
  Departures : PMIOPort  Port=2  Side=Right
  WIP_samples : Outport
  WIP_average : Outport  Port=2
  CT_samples : Outport  Port=3
  CT_average : Outport  Port=4
  TH_samples : Outport  Port=5
  TH_average : Outport  Port=6
  Util_average : Outport  Port=7
  Avail_average : Outport  Port=8
  wires:
  ComputeUandA/2(Avail_average) -> Avail_average/1
  ComputeUandA/1(Util_average) -> Util_average/1
  GG1Workstation_FailuresAndSetups/8(nInProcServer) -> ComputeUandA/3(nInProcServer)
  GG1Workstation_FailuresAndSetups/7(nInFailOrSetupServer) -> ComputeUandA/2(nInFailServer)
  RandomNumbers_SetupTimes/1 -> GG1Workstation_FailuresAndSetups/5(SetupTime)
  RandomNumbers_CountUntilSetup/1 -> GG1Workstation_FailuresAndSetups/4(CountUntilSetup)
  RandomNumbers_TimeToRepair/1 -> GG1Workstation_FailuresAndSetups/3(TimeToRepair)
  RandomNumbers_TimeUntilFailure/1 -> GG1Workstation_FailuresAndSetups/2(TimeUntilFailure)
  ComputeTH/2(TH_samples) -> TH_samples/1
  ComputeTH/1(TH_average) -> TH_average/1
  Clock/1 -> ComputeUandA/1(CurrentTime), ComputeTH/1(CurrentTime), ComputeWIP/3(CurrentTime)
  GG1Workstation_FailuresAndSetups/1(nArrivals) -> ComputeWIP/1(nArrivals)
  ComputeWIP/2(WIP_average) -> WIP_average/1
  ComputeWIP/1(WIP_samples) -> WIP_samples/1
  GG1Workstation_FailuresAndSetups/4(CT_average) -> CT_average/1
  GG1Workstation_FailuresAndSetups/3(CT_samples) -> CT_samples/1
  GG1Workstation_FailuresAndSetups/2(nDepartures) -> ComputeTH/2(nDepartures), ComputeWIP/2(nDepartures)
  RandomNumbers_ProcessingTimes/1 -> GG1Workstation_FailuresAndSetups/1(ProcessingTime)
  connections:
  Arrivals/RConn1 -- GG1Workstation_FailuresAndSetups/LConn1
  GG1Workstation_FailuresAndSetups/RConn1 -- Departures/RConn1

== system ProdSys_MakeToStockPULL_CONWIP/GG1Workstation_FailuresAndSetups1/ComputeTH ==
  CurrentTime : Inport
  nDepartures : Inport  Port=2
  Derivative : Derivative
  Divide1 : Product  Inputs=/*
  Event to Timed Signal1 : EventToTimedSignal
  TH_average : Outport
  TH_samples : Outport  Port=2
  wires:
  nDepartures/1 -> Event to Timed Signal1/1
  Derivative/1 -> TH_samples/1
  Divide1/1 -> TH_average/1
  Event to Timed Signal1/1 -> Divide1/2, Derivative/1
  CurrentTime/1 -> Divide1/1

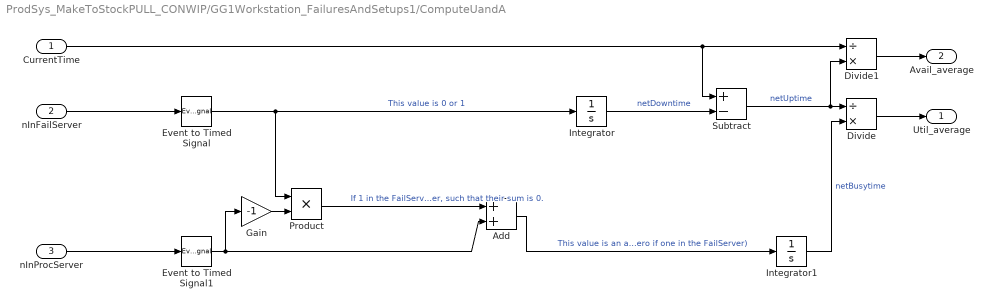
== system ProdSys_MakeToStockPULL_CONWIP/GG1Workstation_FailuresAndSetups1/ComputeUandA ==
  CurrentTime : Inport
  nInFailServer : Inport  Port=2
  nInProcServer : Inport  Port=3
  Add : Sum
  Divide : Product  Inputs=/*
  Divide1 : Product  Inputs=/*
  Event to Timed Signal : EventToTimedSignal
  Event to Timed Signal1 : EventToTimedSignal
  Gain : Gain  Gain=-1
  Integrator : Integrator
  Integrator1 : Integrator
  Product : Product
  Subtract : Sum  Inputs=+-
  Util_average : Outport
  Avail_average : Outport  Port=2
  wires:
  Divide1/1 -> Avail_average/1
  Event to Timed Signal1/1 -> Gain/1, Add/2
  Add/1 -> Integrator1/1  "This value is an adjusted number in the ProcServer (zero if one in the FailServer)"
  Product/1 -> Add/1  "If 1 in the FailServer, then this value should be negative the number in the ProcServer, such that their sum is 0."
  Gain/1 -> Product/2
  Integrator1/1 -> Divide/2  "netBusytime"
  Subtract/1 -> Divide1/2, Divide/1  "netUptime"
  Divide/1 -> Util_average/1
  CurrentTime/1 -> Divide1/1, Subtract/1
  Integrator/1 -> Subtract/2  "netDowntime"
  nInProcServer/1 -> Event to Timed Signal1/1
  nInFailServer/1 -> Event to Timed Signal/1
  Event to Timed Signal/1 -> Product/1, Integrator/1  "This value is 0 or 1"

== system ProdSys_MakeToStockPULL_CONWIP/GG1Workstation_FailuresAndSetups1/ComputeWIP ==
  nArrivals : Inport
  nDepartures : Inport  Port=2
  CurrentTime : Inport  Port=3
  Divide : Product  Inputs=*/
  Event to Timed Signal : EventToTimedSignal
  Integrator : Integrator
  Subtract : Sum  Inputs=+-
  WIP_samples : Outport
  WIP_average : Outport  Port=2
  wires:
  CurrentTime/1 -> Divide/2
  nDepartures/1 -> Subtract/2
  nArrivals/1 -> Subtract/1
  Integrator/1 -> Divide/1
  Divide/1 -> WIP_average/1
  Event to Timed Signal/1 -> Integrator/1
  Subtract/1 -> Event to Timed Signal/1, WIP_samples/1

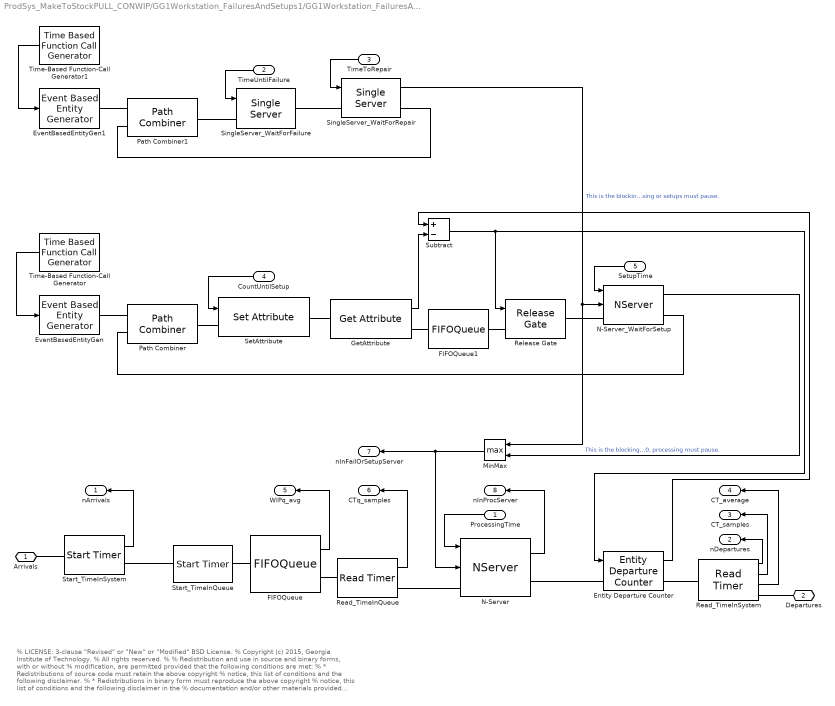
== system ProdSys_MakeToStockPULL_CONWIP/GG1Workstation_FailuresAndSetups1/GG1Workstation_FailuresAndSetups ==
  note: % LICENSE: 3-clause "Revised" or "New" or "Modified" BSD License.
      | % Copyright (c) 2015, Georgia Institute of Technology.
      | % All rights reserved.
      | %
      | % Redistribution and use in source and binary forms, with or without
      | % modification, are permitted provided that the following conditions are met:
      | % * Redistributions of source code must retain the above copyright
      | % notice, this list of conditions and the following disclaimer.
      | % * Redistributions in binary form must reproduce the above copyright
      | % notice, this list of conditions and the following disclaimer in the
      | % documentation and/or other materials provided with the distribution.
      | % * Neither the name of the Georgia Institute of Technology nor the
      | % names of its contributors may be used to endorse or promote products
      | % derived from this software without specific prior written permission.
      | %
      | % THIS SOFTWARE IS PROVIDED BY THE COPYRIGHT HOLDERS AND CONTRIBUTORS "AS IS" AND
      | % ANY EXPRESS OR IMPLIED WARRANTIES, INCLUDING, BUT NOT LIMITED TO, THE IMPLIED
      | % WARRANTIES OF MERCHANTABILITY AND FITNESS FOR A PARTICULAR PURPOSE ARE
      | % DISCLAIMED. IN NO EVENT SHALL THE GEORGIA INSTITUTE OF TECHNOLOGY BE LIABLE FOR
      | % ANY DIRECT, INDIRECT, INCIDENTAL, SPECIAL, EXEMPLARY, OR CONSEQUENTIAL DAMAGES
      | % (INCLUDING, BUT NOT LIMITED TO, PROCUREMENT OF SUBSTITUTE GOODS OR SERVICES;
      | % LOSS OF USE, DATA, OR PROFITS; OR BUSINESS INTERRUPTION) HOWEVER CAUSED AND
      | % ON ANY THEORY OF LIABILITY, WHETHER IN CONTRACT, STRICT LIABILITY, OR TORT
      | % (INCLUDING NEGLIGENCE OR OTHERWISE) ARISING IN ANY WAY OUT OF THE USE OF THIS
      | % SOFTWARE, EVEN IF ADVISED OF THE POSSIBILITY OF SUCH DAMAGE.
  ProcessingTime : Inport
  TimeUntilFailure : Inport  Port=2
  TimeToRepair : Inport  Port=3
  CountUntilSetup : Inport  Port=4
  SetupTime : Inport  Port=5
  Entity Departure Counter : EntityDepartureCounter  NumberDepartedToSignal=on  NumberDepartedToAttribute=off  CounterResetTypeOption=Trigger from port tr
  EventBasedEntityGen : EventBasedEntityGenerator  GenerateEntitiesUpon=Function call from port fcn
  EventBasedEntityGen1 : EventBasedEntityGenerator  GenerateEntitiesUpon=Function call from port fcn
  FIFOQueue : FIFOQueue  Capacity=Capacity  StatAverageQueueLength=on
      settings: OutputPortMap=o3
  FIFOQueue1 : FIFOQueue  Capacity=Inf
  GetAttribute : GetAttribute  AttributeName=CountUntilSetup  EvaluatedDefaultAttributeValue={ []}
      settings: OutputPortMap=o1
  MinMax : MinMax  Function=max  Inputs=2
  N-Server : NServer  NumberOfServers=1  ServiceTimeFrom=Signal port t  AllowServiceControl=on  BlockWhileSignalOn=on  StatNumberInBlock=on
      settings: InputPortMap=u0,u1  OutputPortMap=o1
  N-Server_WaitForSetup : NServer  NumberOfServers=1  ServiceTimeFrom=Signal port t  AllowServiceControl=on  BlockWhileSignalOn=on  StatNumberInBlock=on
      settings: InputPortMap=u0,u1  OutputPortMap=o1
  Path Combiner : PathCombiner  NumberInputPorts=2
  Path Combiner1 : PathCombiner  NumberInputPorts=2
  Read_TimeInQueue : ReadTimer  TimerTag=TimeInQueue  StatTimeElapsed=on
      settings: OutputPortMap=o2
  Read_TimeInSystem : ReadTimer  TimerTag=TimeInSystem  StatNumberDeparted=on  StatTimeElapsed=on  StatAverageTimeElapsed=on
      settings: OutputPortMap=o0,o2,o3
  Release Gate : ReleaseGate  OpenGateUpon=Trigger from port tr
  SetAttribute : SetAttribute  AttributeName=CountUntilSetup  AttributeFrom=Signal port  EvaluatedAttributeValue={ []}
  SingleServer_WaitForFailure : SingleServer  ServiceTimeFrom=Signal port t  AttributeName=TimeUntilFailure
  SingleServer_WaitForRepair : SingleServer  ServiceTimeFrom=Signal port t  AttributeName=TimeToRepair  StatNumberInBlock=on
      settings: OutputPortMap=o1
  Start_TimeInQueue : StartTimer  TimerTag=TimeInQueue  TimerStartedOption=Restart
  Start_TimeInSystem : StartTimer  TimerTag=TimeInSystem  TimerStartedOption=Restart  StatNumberDeparted=on
  Subtract : Sum  Inputs=+-
  Time-Based Function-Call Generator : TimeBasedFunctionCallGenerator  EventGenerationMode=Only at simulation start
  Time-Based Function-Call Generator1 : TimeBasedFunctionCallGenerator  EventGenerationMode=Only at simulation start
  Arrivals : PMIOPort  Port=1  Side=Left
  Departures : PMIOPort  Port=2  Side=Right
  nArrivals : Outport
  nDepartures : Outport  Port=2
  CT_samples : Outport  Port=3
  CT_average : Outport  Port=4
  WIPq_avg : Outport  Port=5
  CTq_samples : Outport  Port=6
  nInFailOrSetupServer : Outport  Port=7
  nInProcServer : Outport  Port=8
  wires:
  MinMax/1 -> N-Server/2, nInFailOrSetupServer/1
  N-Server_WaitForSetup/1 -> MinMax/2  "This is the blocking signal from setups.  When >0, processing must pause."
  SingleServer_WaitForRepair/1 -> N-Server_WaitForSetup/2, MinMax/1  "This is the blocking signal from failures. When >0, processing or setups must pause."
  TimeUntilFailure/1 -> SingleServer_WaitForFailure/1
  TimeToRepair/1 -> SingleServer_WaitForRepair/1
  Time-Based Function-Call Generator1/1 -> EventBasedEntityGen1/1
  SetupTime/1 -> N-Server_WaitForSetup/1
  N-Server/1 -> nInProcServer/1
  Entity Departure Counter/1 -> Subtract/1
  GetAttribute/1 -> Subtract/2
  Subtract/1 -> Entity Departure Counter/1, Release Gate/1
  CountUntilSetup/1 -> SetAttribute/1
  Time-Based Function-Call Generator/1 -> EventBasedEntityGen/1
  Read_TimeInSystem/3 -> CT_average/1
  ProcessingTime/1 -> N-Server/1
  Read_TimeInSystem/1 -> nDepartures/1
  Start_TimeInSystem/1 -> nArrivals/1
  FIFOQueue/1 -> WIPq_avg/1
  Read_TimeInQueue/1 -> CTq_samples/1
  Read_TimeInSystem/2 -> CT_samples/1
  connections:
  Path Combiner1/RConn1 -- SingleServer_WaitForFailure/LConn1
  EventBasedEntityGen1/RConn1 -- Path Combiner1/LConn1
  SingleServer_WaitForRepair/LConn1 -- SingleServer_WaitForFailure/RConn1
  Path Combiner1/LConn2 -- SingleServer_WaitForRepair/RConn1
  SetAttribute/RConn1 -- GetAttribute/LConn1
  FIFOQueue1/RConn1 -- Release Gate/LConn1
  N-Server_WaitForSetup/LConn1 -- Release Gate/RConn1
  FIFOQueue1/LConn1 -- GetAttribute/RConn1
  Entity Departure Counter/RConn1 -- Read_TimeInSystem/LConn1
  N-Server/RConn1 -- Entity Departure Counter/LConn1
  Path Combiner/LConn2 -- N-Server_WaitForSetup/RConn1
  EventBasedEntityGen/RConn1 -- Path Combiner/LConn1
  Path Combiner/RConn1 -- SetAttribute/LConn1
  Start_TimeInQueue/RConn1 -- FIFOQueue/LConn1
  Read_TimeInQueue/RConn1 -- N-Server/LConn1
  Read_TimeInSystem/RConn1 -- Departures/RConn1
  Start_TimeInSystem/RConn1 -- Start_TimeInQueue/LConn1
  FIFOQueue/RConn1 -- Read_TimeInQueue/LConn1
  Arrivals/RConn1 -- Start_TimeInSystem/LConn1

== system ProdSys_MakeToStockPULL_CONWIP/GG1Workstation_FailuresAndSetups2/ComputeTH ==
  CurrentTime : Inport
  nDepartures : Inport  Port=2
  Derivative : Derivative
  Divide1 : Product  Inputs=/*
  Event to Timed Signal1 : EventToTimedSignal
  TH_average : Outport
  TH_samples : Outport  Port=2
  wires:
  nDepartures/1 -> Event to Timed Signal1/1
  Derivative/1 -> TH_samples/1
  Divide1/1 -> TH_average/1
  Event to Timed Signal1/1 -> Divide1/2, Derivative/1
  CurrentTime/1 -> Divide1/1

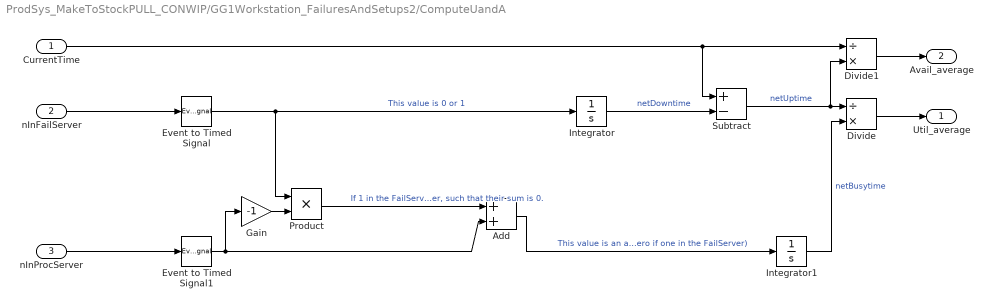
== system ProdSys_MakeToStockPULL_CONWIP/GG1Workstation_FailuresAndSetups2/ComputeUandA ==
  CurrentTime : Inport
  nInFailServer : Inport  Port=2
  nInProcServer : Inport  Port=3
  Add : Sum
  Divide : Product  Inputs=/*
  Divide1 : Product  Inputs=/*
  Event to Timed Signal : EventToTimedSignal
  Event to Timed Signal1 : EventToTimedSignal
  Gain : Gain  Gain=-1
  Integrator : Integrator
  Integrator1 : Integrator
  Product : Product
  Subtract : Sum  Inputs=+-
  Util_average : Outport
  Avail_average : Outport  Port=2
  wires:
  Divide1/1 -> Avail_average/1
  Event to Timed Signal1/1 -> Gain/1, Add/2
  Add/1 -> Integrator1/1  "This value is an adjusted number in the ProcServer (zero if one in the FailServer)"
  Product/1 -> Add/1  "If 1 in the FailServer, then this value should be negative the number in the ProcServer, such that their sum is 0."
  Gain/1 -> Product/2
  Integrator1/1 -> Divide/2  "netBusytime"
  Subtract/1 -> Divide1/2, Divide/1  "netUptime"
  Divide/1 -> Util_average/1
  CurrentTime/1 -> Divide1/1, Subtract/1
  Integrator/1 -> Subtract/2  "netDowntime"
  nInProcServer/1 -> Event to Timed Signal1/1
  nInFailServer/1 -> Event to Timed Signal/1
  Event to Timed Signal/1 -> Product/1, Integrator/1  "This value is 0 or 1"

== system ProdSys_MakeToStockPULL_CONWIP/GG1Workstation_FailuresAndSetups2/ComputeWIP ==
  nArrivals : Inport
  nDepartures : Inport  Port=2
  CurrentTime : Inport  Port=3
  Divide : Product  Inputs=*/
  Event to Timed Signal : EventToTimedSignal
  Integrator : Integrator
  Subtract : Sum  Inputs=+-
  WIP_samples : Outport
  WIP_average : Outport  Port=2
  wires:
  CurrentTime/1 -> Divide/2
  nDepartures/1 -> Subtract/2
  nArrivals/1 -> Subtract/1
  Integrator/1 -> Divide/1
  Divide/1 -> WIP_average/1
  Event to Timed Signal/1 -> Integrator/1
  Subtract/1 -> Event to Timed Signal/1, WIP_samples/1
